simulink model "Diagnostics"  (R2022a)
settings: Solver=VariableStepAuto  StartTime=0.0  StopTime=10.0  RelTol=1e-3
settings Model: Creator=maxju  LastModifiedBy=maxju

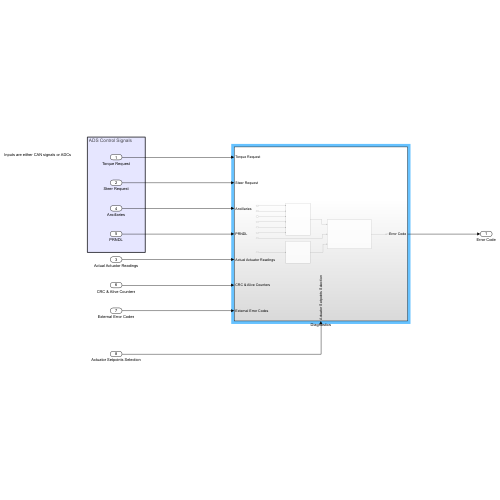
[thumbnail: Simulink's stored preview of the top-level diagram]
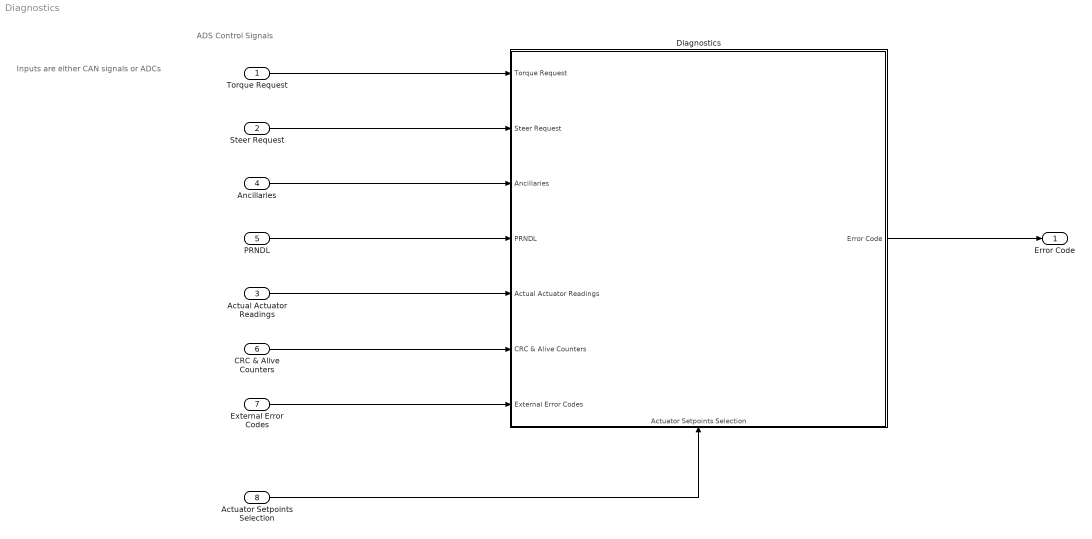
== system Diagnostics ==
  note: Inputs are either CAN signals or ADCs
  note: ADS Control Signals
  Torque Request : Inport
  Steer Request : Inport  Port=2
  Actual Actuator Readings : Inport  Port=3
  Ancillaries : Inport  Port=4
  PRNDL : Inport  Port=5
  CRC & Alive Counters : Inport  Port=6
  External Error Codes : Inport  Port=7
  Actuator Setpoints Selection : Inport  Port=8
  Diagnostics : Subsystem
      settings: PortSchema="{\"entries\":[{\"content\":{\"sides\":[{\"content\":{\"connectorIds\":[\"In1\",\"In2\",\"In3\",\"In4\",\"In5\",\"In6\",\"In7\"]},\"type\":\"ConnectorPlacement.EquallySpacedRectSide\",\"uuid\":\"cd615367-173d-41ff-a4ef-5bcb12e49810\"},{\"content\":{\"connectorIds\":[\"Out1\"],\"side\":\"RIGHT\"},\"type\":\"ConnectorPlacement.EquallySpacedRectSide\",\"uuid\":\"0aa0a36e-e2a8-44d5-a6b9-a78be9d5a0f5\"},{\"content\":{\"connectorIds\":[],\"side\":\"TOP\"},\"type\":\"ConnectorPlacement.EquallySpacedRectSide\",\"uuid\":\"fb7d50c9-14bf-43be-90b1-c2ef3f9c74c3\"},{\"content\":{\"connectorIds\":[\"In8\"],\"side\":\"BOTTOM\"},\"type\":\"ConnectorPlacement.EquallySpacedRectSide\",\"uuid\":\"fc955ed2-3c68-4ea9-8c8c-8c5f23f5e740\"}]},\"type\":\"ConnectorPlacement.EquallySpacedConnector\",\"uuid\":\"6fbd2339-9d8b-4f86-88be-085d341f8c1a\"}],\"packageUris\":[\"http://schema.mathworks.com/mf0/Connector/R2020b\"],\"version\":\"1.0\"}"
  Error Code : Outport
  wires:
  Torque Request/1 -> Diagnostics/1(Torque Request)
  Steer Request/1 -> Diagnostics/2(Steer Request)
  Ancillaries/1 -> Diagnostics/3(Ancillaries)
  Actual Actuator Readings/1 -> Diagnostics/5(Actual Actuator Readings)
  PRNDL/1 -> Diagnostics/4(PRNDL)
  CRC & Alive Counters/1 -> Diagnostics/6(CRC & Alive Counters)
  External Error Codes/1 -> Diagnostics/7(External Error Codes)
  Actuator Setpoints Selection/1 -> Diagnostics/8(Actuator Setpoints Selection)
  Diagnostics/1(Error Code) -> Error Code/1

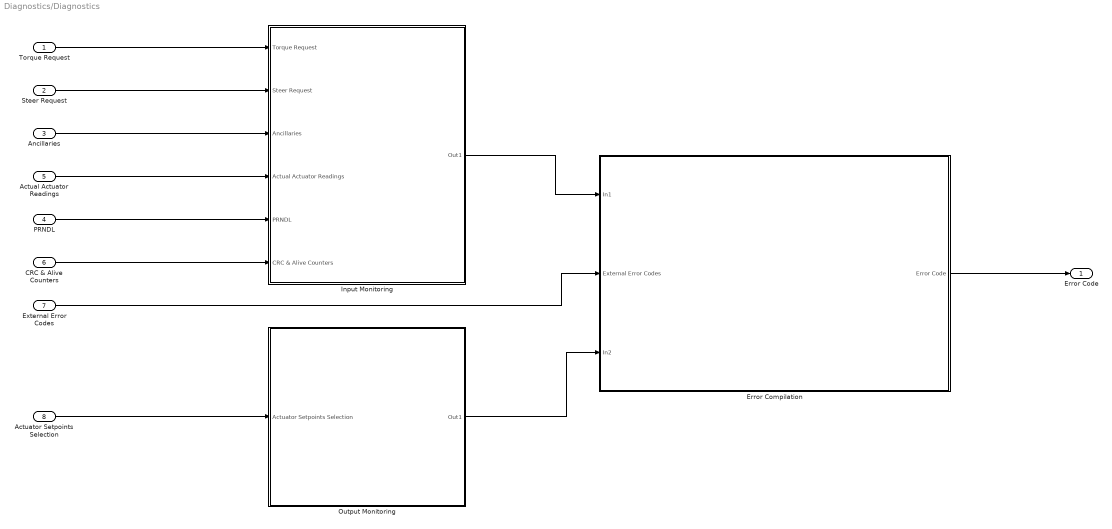
== system Diagnostics/Diagnostics ==
  Torque Request : Inport
  Steer Request : Inport  Port=2
  Ancillaries : Inport  Port=3
  PRNDL : Inport  Port=4
  Actual Actuator Readings : Inport  Port=5
  CRC & Alive Counters : Inport  Port=6
  External Error Codes : Inport  Port=7
  Actuator Setpoints Selection : Inport  Port=8
  Error Compilation : Subsystem
  Input Monitoring : Subsystem
  Output Monitoring : Subsystem
  Error Code : Outport
  wires:
  Error Compilation/1(Error Code) -> Error Code/1
  Input Monitoring/1(Out1) -> Error Compilation/1(In1)
  Output Monitoring/1(Out1) -> Error Compilation/3(In2)
  External Error Codes/1 -> Error Compilation/2(External Error Codes)
  Torque Request/1 -> Input Monitoring/1(Torque Request)
  Steer Request/1 -> Input Monitoring/2(Steer Request)
  Ancillaries/1 -> Input Monitoring/3(Ancillaries)
  Actual Actuator Readings/1 -> Input Monitoring/4(Actual Actuator Readings)
  PRNDL/1 -> Input Monitoring/5(PRNDL)
  CRC & Alive Counters/1 -> Input Monitoring/6(CRC & Alive Counters)
  Actuator Setpoints Selection/1 -> Output Monitoring/1(Actuator Setpoints Selection)

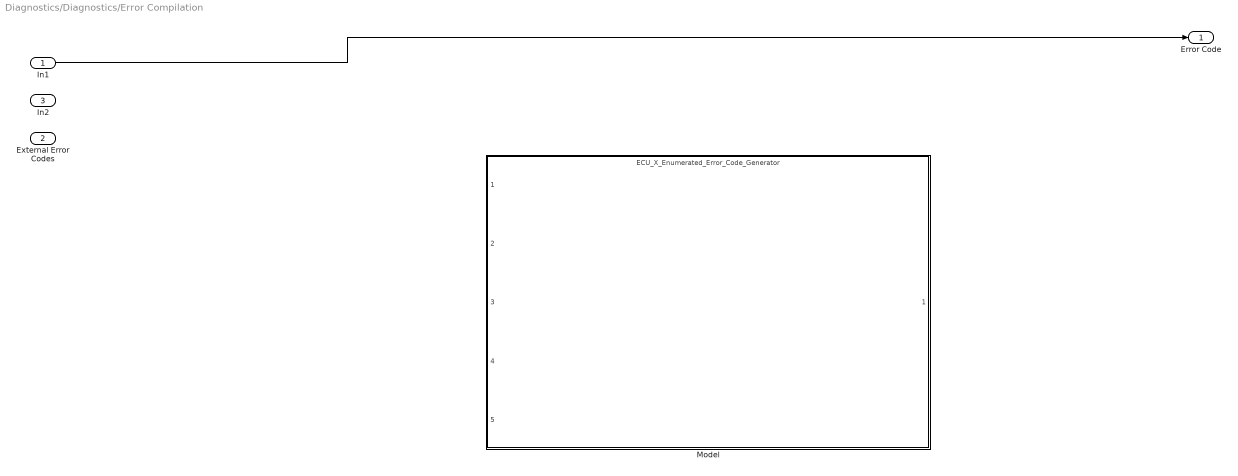
== system Diagnostics/Diagnostics/Error Compilation ==
  In1 : Inport
  External Error Codes : Inport  Port=2
  In2 : Inport  Port=3
  Model : ModelReference  ModelNameDialog=ECU_X_Enumerated_Error_Code_Generator.slx  SimulationMode=Normal  ModelReferenceVersion=1.13
  Error Code : Outport
  wires:
  In1/1 -> Error Code/1

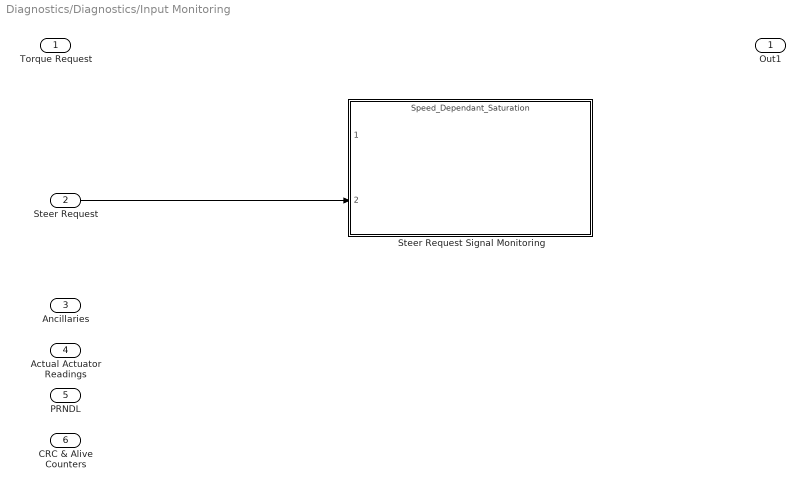
== system Diagnostics/Diagnostics/Input Monitoring ==
  Torque Request : Inport
  Steer Request : Inport  Port=2
  Ancillaries : Inport  Port=3
  Actual Actuator Readings : Inport  Port=4
  PRNDL : Inport  Port=5
  CRC & Alive Counters : Inport  Port=6
  Steer Request Signal Monitoring : ModelReference  ModelNameDialog=Speed_Dependant_Saturation.slx  SimulationMode=Normal  ModelReferenceVersion=1.5
  Out1 : Outport
  wires:
  Steer Request/1 -> Steer Request Signal Monitoring/2

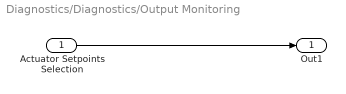
== system Diagnostics/Diagnostics/Output Monitoring ==
  Actuator Setpoints Selection : Inport
  Out1 : Outport
  wires:
  Actuator Setpoints Selection/1 -> Out1/1
